simulink model "SchemaControlloDecentralizzatoSmartSixR2013a"  (Simulink 8.7)
settings: Solver=ode45  StartTime=0.0  StopTime=t(end)+Tf  FixedStep=T  MaxStep=T  RelTol=1e-3
PreLoadFcn:
  | initFunction
InitFcn:
  | initFunction
StopFcn:
  | cd ..
  | 
  | figure
  | subplot(31,1)
  | plot(err_q.data(1:50))
  | subplot(312)
  | plot(err_dq.data(1:50))
  | subplot(313)
  | plot(err_ddq.data(1:50))
values from neighbouring files (symbols this model uses):
  FM = Kr^-1*Fv*Kr^-1    [initFunction.m]
  Im = Kr^-1*Bconst*Kr^-1    [initFunction.m]
  KCA = [586.881582263 0 0 0 0 0 0 566.981582263 0 0 0 0 ... (36 elements, 6x6)]    [KCA.mat]
  KCP = [63 0 0 0 0 0 0 63 0 0 0 0 ... (36 elements, 6x6)]    [KCP.mat]
  KCV = [315.577034284 0 0 0 0 0 0 325.715347644 0 0 0 0 ... (36 elements, 6x6)]    [KCV.mat]    (also in initFunction.m = KCV*rKCV^-1)
  KM = [0.0232558139535 0 0 0 0 0 0 0.0158982511924 0 0 0 0 ... (36 elements, 6x6)]    [KM.mat]
  Kr = diag(kr)    [ParametriMotori.m]
  Kt = diag(kt)    [ParametriMotori.m]
  KTA = [1 0 0 0 0 0 0 1 0 0 0 0 ... (36 elements, 6x6)]    [KTA.mat]
  KTP = [1 0 0 0 0 0 0 1 0 0 0 0 ... (36 elements, 6x6)]    [KTP.mat]
  KTV = [1 0 0 0 0 0 0 1 0 0 0 0 ... (36 elements, 6x6)]    [KTV.mat]
  Kv = diag(kv)    [ParametriMotori.m]
  La = diag(la)    [ParametriMotori.m]
  q0 = q0'    [initFunction.m]
  Ra = diag(ra)    [ParametriMotori.m]
  T = Tf    (= 0.002)    [initFunction.m]
  TCA = [4.96122857983e-05 0 0 0 0 0 0 3.97711481373e-05 0 0 0 0 ... (36 elements, 6x6)]    [TCA.mat]
libraries: simulink x18
(part 2 of 2)

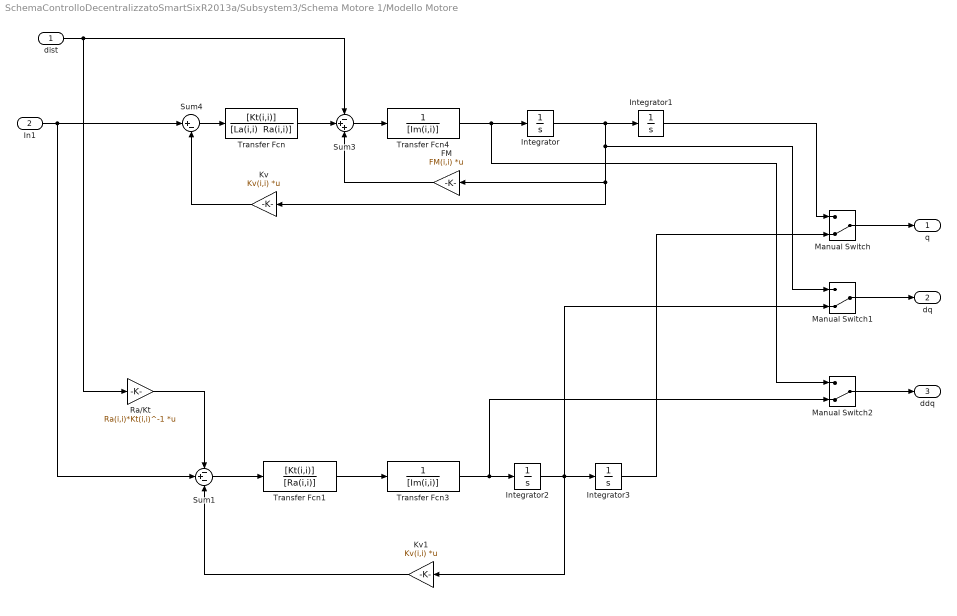
== system SchemaControlloDecentralizzatoSmartSixR2013a/Subsystem3/Schema Motore 1/Modello Motore ==
  dist : Inport
  In1 : Inport  Port=2
  FM : Gain  Gain=FM(i,i)  Multiplication=Matrix(K*u)
  Integrator : Integrator
  Integrator1 : Integrator  InitialCondition=q0(i)
  Integrator2 : Integrator
  Integrator3 : Integrator  InitialCondition=q0(i)
  Kv : Gain  Gain=Kv(i,i)  Multiplication=Matrix(K*u)
  Kv1 : Gain  Gain=Kv(i,i)  Multiplication=Matrix(K*u)
  Manual Switch : ManualSwitch  CurrentSetting=0
  Manual Switch1 : ManualSwitch  CurrentSetting=0
  Manual Switch2 : ManualSwitch  CurrentSetting=0
  Ra/Kt : Gain  Gain=Ra(i,i)*Kt(i,i)^-1  Multiplication=Matrix(K*u)
  Sum1 : Sum  Inputs=-+-
  Sum3 : Sum  Inputs=-++
  Sum4 : Sum  Inputs=|+-
  Transfer Fcn : TransferFcn  Numerator=[Kt(i,i)]  Denominator="[La(i,i)  Ra(i,i)]"
  Transfer Fcn1 : TransferFcn  Numerator=[Kt(i,i)]  Denominator=[Ra(i,i)]
  Transfer Fcn3 : TransferFcn  Denominator=[Im(i,i)]
  Transfer Fcn4 : TransferFcn  Denominator=[Im(i,i)]
  q : Outport
  dq : Outport  Port=2
  ddq : Outport  Port=3
  wires:
  Manual Switch2/1 -> ddq/1
  Manual Switch1/1 -> dq/1
  Manual Switch/1 -> q/1
  Integrator/1 -> Kv/1, FM/1, Manual Switch1/1, Integrator1/1
  Kv/1 -> Sum4/2
  In1/1 -> Sum1/2, Sum4/1
  Sum4/1 -> Transfer Fcn/1
  Transfer Fcn/1 -> Sum3/2
  FM/1 -> Sum3/3
  Integrator1/1 -> Manual Switch/1
  dist/1 -> Ra/Kt/1, Sum3/1
  Ra/Kt/1 -> Sum1/1
  Sum1/1 -> Transfer Fcn1/1
  Transfer Fcn1/1 -> Transfer Fcn3/1
  Transfer Fcn3/1 -> Manual Switch2/2, Integrator2/1
  Integrator2/1 -> Manual Switch1/2, Kv1/1, Integrator3/1
  Kv1/1 -> Sum1/3
  Integrator3/1 -> Manual Switch/2
  Sum3/1 -> Transfer Fcn4/1
  Transfer Fcn4/1 -> Manual Switch2/1, Integrator/1

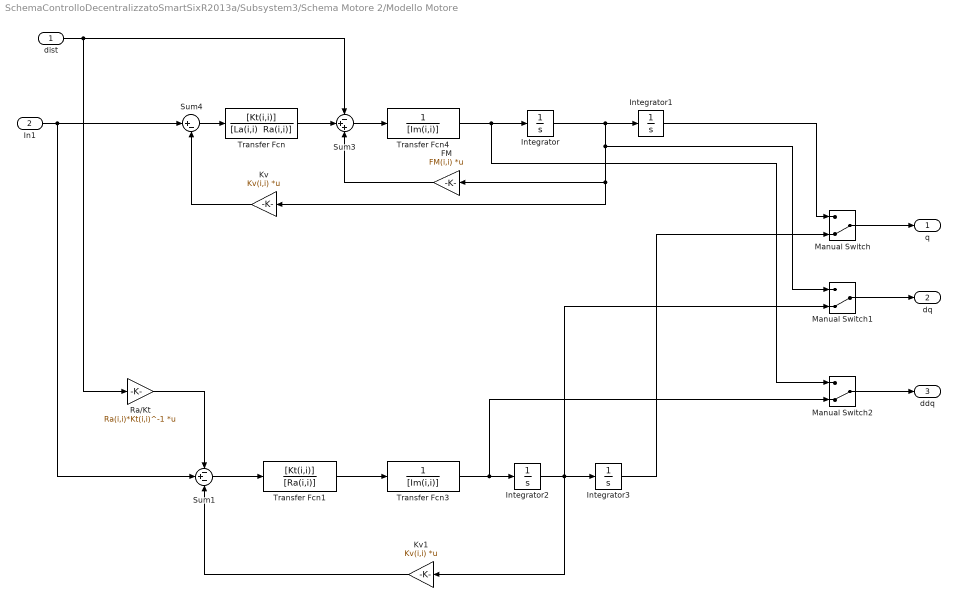
== system SchemaControlloDecentralizzatoSmartSixR2013a/Subsystem3/Schema Motore 2/Modello Motore ==
  dist : Inport
  In1 : Inport  Port=2
  FM : Gain  Gain=FM(i,i)  Multiplication=Matrix(K*u)
  Integrator : Integrator
  Integrator1 : Integrator  InitialCondition=q0(i)
  Integrator2 : Integrator
  Integrator3 : Integrator  InitialCondition=q0(i)
  Kv : Gain  Gain=Kv(i,i)  Multiplication=Matrix(K*u)
  Kv1 : Gain  Gain=Kv(i,i)  Multiplication=Matrix(K*u)
  Manual Switch : ManualSwitch  CurrentSetting=0
  Manual Switch1 : ManualSwitch  CurrentSetting=0
  Manual Switch2 : ManualSwitch  CurrentSetting=0
  Ra/Kt : Gain  Gain=Ra(i,i)*Kt(i,i)^-1  Multiplication=Matrix(K*u)
  Sum1 : Sum  Inputs=-+-
  Sum3 : Sum  Inputs=-++
  Sum4 : Sum  Inputs=|+-
  Transfer Fcn : TransferFcn  Numerator=[Kt(i,i)]  Denominator="[La(i,i)  Ra(i,i)]"
  Transfer Fcn1 : TransferFcn  Numerator=[Kt(i,i)]  Denominator=[Ra(i,i)]
  Transfer Fcn3 : TransferFcn  Denominator=[Im(i,i)]
  Transfer Fcn4 : TransferFcn  Denominator=[Im(i,i)]
  q : Outport
  dq : Outport  Port=2
  ddq : Outport  Port=3
  wires:
  Manual Switch2/1 -> ddq/1
  Manual Switch1/1 -> dq/1
  Manual Switch/1 -> q/1
  Integrator/1 -> Kv/1, FM/1, Manual Switch1/1, Integrator1/1
  Kv/1 -> Sum4/2
  In1/1 -> Sum1/2, Sum4/1
  Sum4/1 -> Transfer Fcn/1
  Transfer Fcn/1 -> Sum3/2
  FM/1 -> Sum3/3
  Integrator1/1 -> Manual Switch/1
  dist/1 -> Ra/Kt/1, Sum3/1
  Ra/Kt/1 -> Sum1/1
  Sum1/1 -> Transfer Fcn1/1
  Transfer Fcn1/1 -> Transfer Fcn3/1
  Transfer Fcn3/1 -> Manual Switch2/2, Integrator2/1
  Integrator2/1 -> Manual Switch1/2, Kv1/1, Integrator3/1
  Kv1/1 -> Sum1/3
  Integrator3/1 -> Manual Switch/2
  Sum3/1 -> Transfer Fcn4/1
  Transfer Fcn4/1 -> Manual Switch2/1, Integrator/1

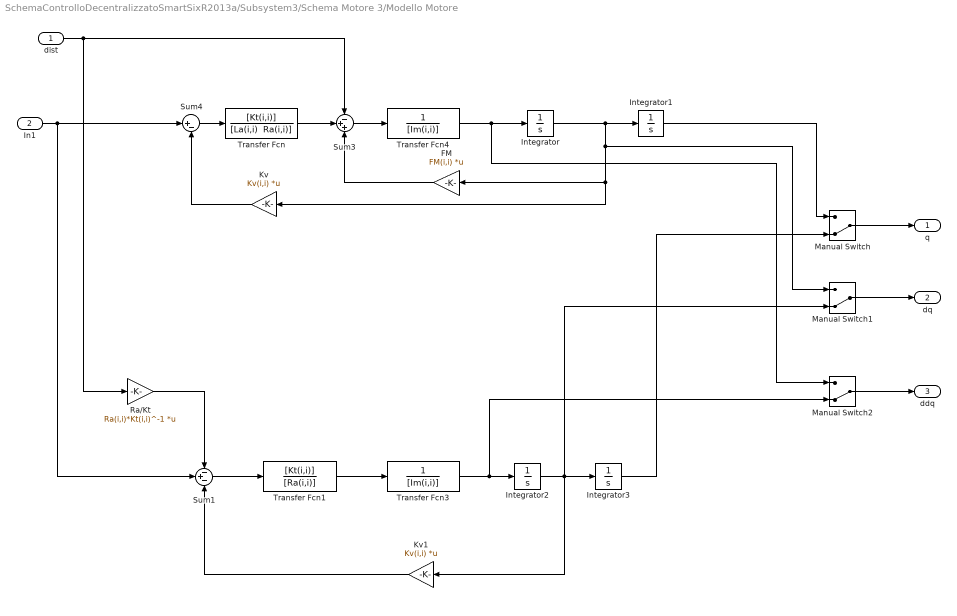
== system SchemaControlloDecentralizzatoSmartSixR2013a/Subsystem3/Schema Motore 3/Modello Motore ==
  dist : Inport
  In1 : Inport  Port=2
  FM : Gain  Gain=FM(i,i)  Multiplication=Matrix(K*u)
  Integrator : Integrator
  Integrator1 : Integrator  InitialCondition=q0(i)
  Integrator2 : Integrator
  Integrator3 : Integrator  InitialCondition=q0(i)
  Kv : Gain  Gain=Kv(i,i)  Multiplication=Matrix(K*u)
  Kv1 : Gain  Gain=Kv(i,i)  Multiplication=Matrix(K*u)
  Manual Switch : ManualSwitch  CurrentSetting=0
  Manual Switch1 : ManualSwitch  CurrentSetting=0
  Manual Switch2 : ManualSwitch  CurrentSetting=0
  Ra/Kt : Gain  Gain=Ra(i,i)*Kt(i,i)^-1  Multiplication=Matrix(K*u)
  Sum1 : Sum  Inputs=-+-
  Sum3 : Sum  Inputs=-++
  Sum4 : Sum  Inputs=|+-
  Transfer Fcn : TransferFcn  Numerator=[Kt(i,i)]  Denominator="[La(i,i)  Ra(i,i)]"
  Transfer Fcn1 : TransferFcn  Numerator=[Kt(i,i)]  Denominator=[Ra(i,i)]
  Transfer Fcn3 : TransferFcn  Denominator=[Im(i,i)]
  Transfer Fcn4 : TransferFcn  Denominator=[Im(i,i)]
  q : Outport
  dq : Outport  Port=2
  ddq : Outport  Port=3
  wires:
  Manual Switch2/1 -> ddq/1
  Manual Switch1/1 -> dq/1
  Manual Switch/1 -> q/1
  Integrator/1 -> Kv/1, FM/1, Manual Switch1/1, Integrator1/1
  Kv/1 -> Sum4/2
  In1/1 -> Sum1/2, Sum4/1
  Sum4/1 -> Transfer Fcn/1
  Transfer Fcn/1 -> Sum3/2
  FM/1 -> Sum3/3
  Integrator1/1 -> Manual Switch/1
  dist/1 -> Ra/Kt/1, Sum3/1
  Ra/Kt/1 -> Sum1/1
  Sum1/1 -> Transfer Fcn1/1
  Transfer Fcn1/1 -> Transfer Fcn3/1
  Transfer Fcn3/1 -> Manual Switch2/2, Integrator2/1
  Integrator2/1 -> Manual Switch1/2, Kv1/1, Integrator3/1
  Kv1/1 -> Sum1/3
  Integrator3/1 -> Manual Switch/2
  Sum3/1 -> Transfer Fcn4/1
  Transfer Fcn4/1 -> Manual Switch2/1, Integrator/1

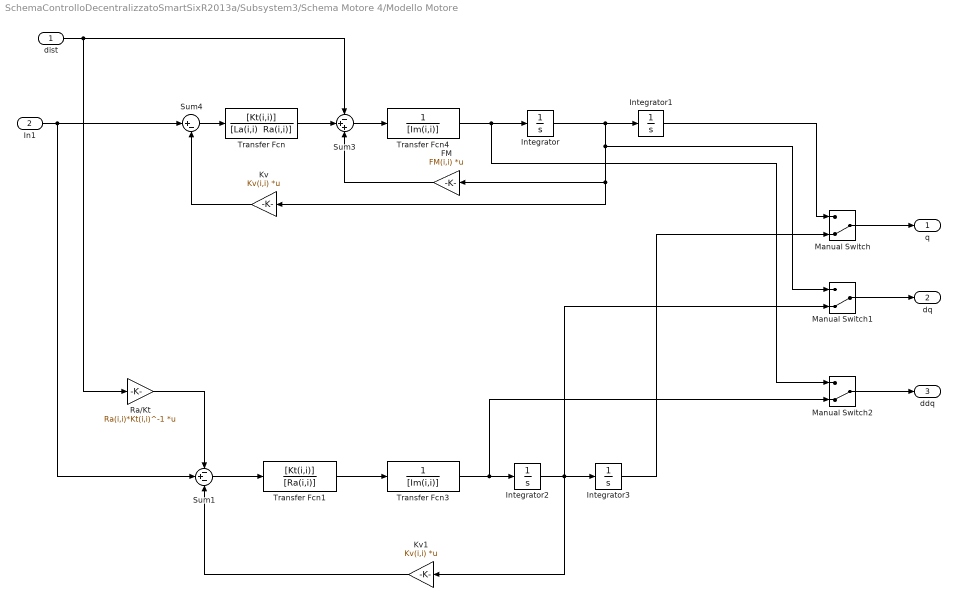
== system SchemaControlloDecentralizzatoSmartSixR2013a/Subsystem3/Schema Motore 4/Modello Motore ==
  dist : Inport
  In1 : Inport  Port=2
  FM : Gain  Gain=FM(i,i)  Multiplication=Matrix(K*u)
  Integrator : Integrator
  Integrator1 : Integrator  InitialCondition=q0(i)
  Integrator2 : Integrator
  Integrator3 : Integrator  InitialCondition=q0(i)
  Kv : Gain  Gain=Kv(i,i)  Multiplication=Matrix(K*u)
  Kv1 : Gain  Gain=Kv(i,i)  Multiplication=Matrix(K*u)
  Manual Switch : ManualSwitch  CurrentSetting=0
  Manual Switch1 : ManualSwitch  CurrentSetting=0
  Manual Switch2 : ManualSwitch  CurrentSetting=0
  Ra/Kt : Gain  Gain=Ra(i,i)*Kt(i,i)^-1  Multiplication=Matrix(K*u)
  Sum1 : Sum  Inputs=-+-
  Sum3 : Sum  Inputs=-++
  Sum4 : Sum  Inputs=|+-
  Transfer Fcn : TransferFcn  Numerator=[Kt(i,i)]  Denominator="[La(i,i)  Ra(i,i)]"
  Transfer Fcn1 : TransferFcn  Numerator=[Kt(i,i)]  Denominator=[Ra(i,i)]
  Transfer Fcn3 : TransferFcn  Denominator=[Im(i,i)]
  Transfer Fcn4 : TransferFcn  Denominator=[Im(i,i)]
  q : Outport
  dq : Outport  Port=2
  ddq : Outport  Port=3
  wires:
  Manual Switch2/1 -> ddq/1
  Manual Switch1/1 -> dq/1
  Manual Switch/1 -> q/1
  Integrator/1 -> Kv/1, FM/1, Manual Switch1/1, Integrator1/1
  Kv/1 -> Sum4/2
  In1/1 -> Sum1/2, Sum4/1
  Sum4/1 -> Transfer Fcn/1
  Transfer Fcn/1 -> Sum3/2
  FM/1 -> Sum3/3
  Integrator1/1 -> Manual Switch/1
  dist/1 -> Ra/Kt/1, Sum3/1
  Ra/Kt/1 -> Sum1/1
  Sum1/1 -> Transfer Fcn1/1
  Transfer Fcn1/1 -> Transfer Fcn3/1
  Transfer Fcn3/1 -> Manual Switch2/2, Integrator2/1
  Integrator2/1 -> Manual Switch1/2, Kv1/1, Integrator3/1
  Kv1/1 -> Sum1/3
  Integrator3/1 -> Manual Switch/2
  Sum3/1 -> Transfer Fcn4/1
  Transfer Fcn4/1 -> Manual Switch2/1, Integrator/1

== system SchemaControlloDecentralizzatoSmartSixR2013a/Subsystem3/Schema Motore 5/Modello Motore ==
  dist : Inport
  In1 : Inport  Port=2
  FM : Gain  Gain=FM(i,i)  Multiplication=Matrix(K*u)
  Integrator : Integrator
  Integrator1 : Integrator  InitialCondition=q0(i)
  Integrator2 : Integrator
  Integrator3 : Integrator  InitialCondition=q0(i)
  Kv : Gain  Gain=Kv(i,i)  Multiplication=Matrix(K*u)
  Kv1 : Gain  Gain=Kv(i,i)  Multiplication=Matrix(K*u)
  Manual Switch : ManualSwitch  CurrentSetting=0
  Manual Switch1 : ManualSwitch  CurrentSetting=0
  Manual Switch2 : ManualSwitch  CurrentSetting=0
  Ra/Kt : Gain  Gain=Ra(i,i)*Kt(i,i)^-1  Multiplication=Matrix(K*u)
  Sum1 : Sum  Inputs=-+-
  Sum3 : Sum  Inputs=-++
  Sum4 : Sum  Inputs=|+-
  Transfer Fcn : TransferFcn  Numerator=[Kt(i,i)]  Denominator="[La(i,i)  Ra(i,i)]"
  Transfer Fcn1 : TransferFcn  Numerator=[Kt(i,i)]  Denominator=[Ra(i,i)]
  Transfer Fcn3 : TransferFcn  Denominator=[Im(i,i)]
  Transfer Fcn4 : TransferFcn  Denominator=[Im(i,i)]
  q : Outport
  dq : Outport  Port=2
  ddq : Outport  Port=3
  wires:
  Manual Switch2/1 -> ddq/1
  Manual Switch1/1 -> dq/1
  Manual Switch/1 -> q/1
  Integrator/1 -> Kv/1, FM/1, Manual Switch1/1, Integrator1/1
  Kv/1 -> Sum4/2
  In1/1 -> Sum1/2, Sum4/1
  Sum4/1 -> Transfer Fcn/1
  Transfer Fcn/1 -> Sum3/2
  FM/1 -> Sum3/3
  Integrator1/1 -> Manual Switch/1
  dist/1 -> Ra/Kt/1, Sum3/1
  Ra/Kt/1 -> Sum1/1
  Sum1/1 -> Transfer Fcn1/1
  Transfer Fcn1/1 -> Transfer Fcn3/1
  Transfer Fcn3/1 -> Manual Switch2/2, Integrator2/1
  Integrator2/1 -> Manual Switch1/2, Kv1/1, Integrator3/1
  Kv1/1 -> Sum1/3
  Integrator3/1 -> Manual Switch/2
  Sum3/1 -> Transfer Fcn4/1
  Transfer Fcn4/1 -> Manual Switch2/1, Integrator/1

== system SchemaControlloDecentralizzatoSmartSixR2013a/Subsystem3/Schema Motore 6/Modello Motore ==
  dist : Inport
  In1 : Inport  Port=2
  FM : Gain  Gain=FM(i,i)  Multiplication=Matrix(K*u)
  Integrator : Integrator
  Integrator1 : Integrator  InitialCondition=q0(i)
  Integrator2 : Integrator
  Integrator3 : Integrator  InitialCondition=q0(i)
  Kv : Gain  Gain=Kv(i,i)  Multiplication=Matrix(K*u)
  Kv1 : Gain  Gain=Kv(i,i)  Multiplication=Matrix(K*u)
  Manual Switch : ManualSwitch  CurrentSetting=0
  Manual Switch1 : ManualSwitch  CurrentSetting=0
  Manual Switch2 : ManualSwitch  CurrentSetting=0
  Ra/Kt : Gain  Gain=Ra(i,i)*Kt(i,i)^-1  Multiplication=Matrix(K*u)
  Sum1 : Sum  Inputs=-+-
  Sum3 : Sum  Inputs=-++
  Sum4 : Sum  Inputs=|+-
  Transfer Fcn : TransferFcn  Numerator=[Kt(i,i)]  Denominator="[La(i,i)  Ra(i,i)]"
  Transfer Fcn1 : TransferFcn  Numerator=[Kt(i,i)]  Denominator=[Ra(i,i)]
  Transfer Fcn3 : TransferFcn  Denominator=[Im(i,i)]
  Transfer Fcn4 : TransferFcn  Denominator=[Im(i,i)]
  q : Outport
  dq : Outport  Port=2
  ddq : Outport  Port=3
  wires:
  Manual Switch2/1 -> ddq/1
  Manual Switch1/1 -> dq/1
  Manual Switch/1 -> q/1
  Integrator/1 -> Kv/1, FM/1, Manual Switch1/1, Integrator1/1
  Kv/1 -> Sum4/2
  In1/1 -> Sum1/2, Sum4/1
  Sum4/1 -> Transfer Fcn/1
  Transfer Fcn/1 -> Sum3/2
  FM/1 -> Sum3/3
  Integrator1/1 -> Manual Switch/1
  dist/1 -> Ra/Kt/1, Sum3/1
  Ra/Kt/1 -> Sum1/1
  Sum1/1 -> Transfer Fcn1/1
  Transfer Fcn1/1 -> Transfer Fcn3/1
  Transfer Fcn3/1 -> Manual Switch2/2, Integrator2/1
  Integrator2/1 -> Manual Switch1/2, Kv1/1, Integrator3/1
  Kv1/1 -> Sum1/3
  Integrator3/1 -> Manual Switch/2
  Sum3/1 -> Transfer Fcn4/1
  Transfer Fcn4/1 -> Manual Switch2/1, Integrator/1
